simulink model "test_TM1654P"  (R2018b)
settings: Solver=FixedStepAuto  StartTime=0.0  StopTime=30  FixedStep=0.001  RelTol=1e-3
libraries: dspsrcs4 x1
settings Model: Creator=39926  LastModifiedBy=39926

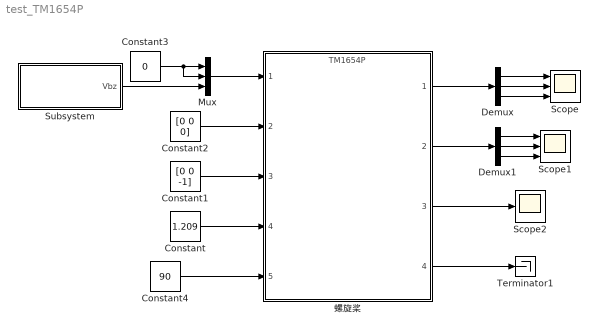
== system test_TM1654P ==
  Constant : Constant  Value=1.209  SampleTime=0
  Constant1 : Constant  Value=[0 0 -1]  SampleTime=0
  Constant2 : Constant  Value=[0 0 0]  SampleTime=0
  Constant3 : Constant  Value=0
  Constant4 : Constant  Value=90
  Demux : Demux  Outputs=3
  Demux1 : Demux  Outputs=3
  Mux : Mux  Inputs=3
  Scope : Scope  NumInputPorts=3
  Scope1 : Scope  NumInputPorts=3
  Scope2 : Scope
  Subsystem : Subsystem
  Terminator1 : Terminator
  螺旋桨 : ModelReference  ModelNameDialog=TM1654P  SimulationMode=Normal  ModelReferenceVersion=1.89
  wires:
  Mux/1 -> 螺旋桨/1
  Constant2/1 -> 螺旋桨/2
  Constant1/1 -> 螺旋桨/3
  Constant/1 -> 螺旋桨/4
  螺旋桨/1 -> Demux/1
  螺旋桨/2 -> Demux1/1
  Constant4/1 -> 螺旋桨/5
  螺旋桨/3 -> Scope2/1
  螺旋桨/4 -> Terminator1/1
  Demux/1 -> Scope/1
  Demux/2 -> Scope/2
  Demux/3 -> Scope/3
  Demux1/1 -> Scope1/1
  Demux1/2 -> Scope1/2
  Demux1/3 -> Scope1/3
  Subsystem/1("Vbz ") -> Mux/3
  Constant3/1 -> Mux/2, Mux/1

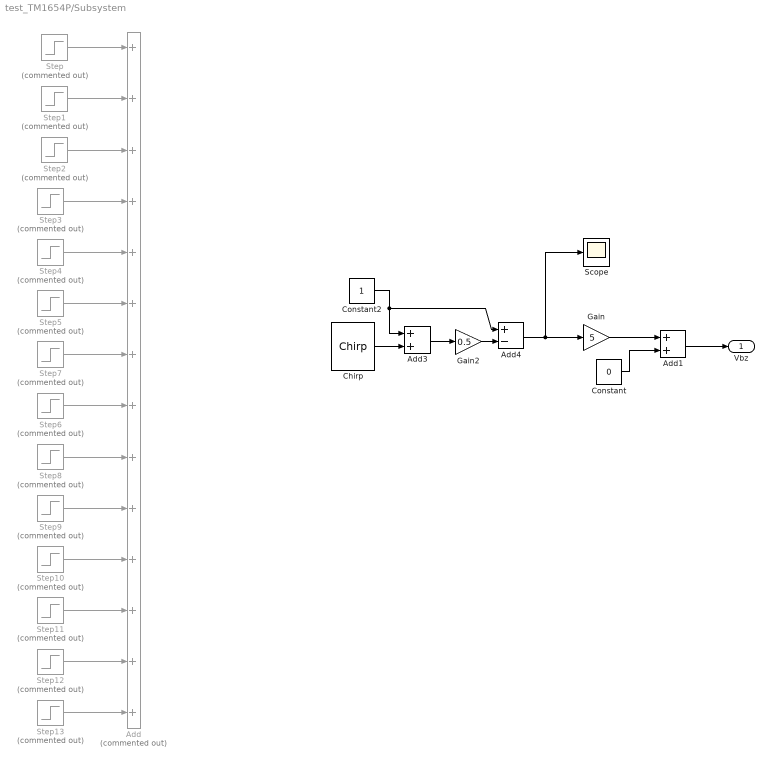
== system test_TM1654P/Subsystem ==
  Add : Sum  Commented=on  Inputs=++++++++++++++
  Add1 : Sum
  Add3 : Sum
  Add4 : Sum  Inputs=+-
  Chirp : dspsrcs4/Chirp  sweep=Linear  mode=Unidirectional  f0=0.1  f1=4  t1=30  Tsweep=30  phase=0  Ts=1/1000  spf=1  datatype=Double  OutputFrames=off
      settings: SourceProductName=DSP System Toolbox
  Constant : Constant  Value=0
  Constant2 : Constant
  Gain : Gain  Gain=5
  Gain2 : Gain  Gain=0.5
  Scope : Scope
  Step : Step  Commented=on  Time=2  After=1/14  SampleTime=0
  Step1 : Step  Commented=on  Time=4  After=1/14  SampleTime=0
  Step10 : Step  Commented=on  Time=22  After=1/14  SampleTime=0
  Step11 : Step  Commented=on  Time=24  After=1/14  SampleTime=0
  Step12 : Step  Commented=on  Time=26  After=1/14  SampleTime=0
  Step13 : Step  Commented=on  Time=28  After=1/14  SampleTime=0
  Step2 : Step  Commented=on  Time=6  After=1/14  SampleTime=0
  Step3 : Step  Commented=on  Time=8  After=1/14  SampleTime=0
  Step4 : Step  Commented=on  Time=10  After=1/14  SampleTime=0
  Step5 : Step  Commented=on  Time=12  After=1/14  SampleTime=0
  Step6 : Step  Commented=on  Time=16  After=1/14  SampleTime=0
  Step7 : Step  Commented=on  Time=14  After=1/14  SampleTime=0
  Step8 : Step  Commented=on  Time=18  After=1/14  SampleTime=0
  Step9 : Step  Commented=on  Time=20  After=1/14  SampleTime=0
  "Vbz " : Outport
  wires:
  Step/1 -> Add/1
  Step1/1 -> Add/2
  Step2/1 -> Add/3
  Step3/1 -> Add/4
  Step4/1 -> Add/5
  Step5/1 -> Add/6
  Step6/1 -> Add/8
  Gain/1 -> Add1/1
  Constant/1 -> Add1/2
  Add1/1 -> "Vbz "/1
  Step7/1 -> Add/7
  Step8/1 -> Add/9
  Step9/1 -> Add/10
  Step10/1 -> Add/11
  Step11/1 -> Add/12
  Step12/1 -> Add/13
  Step13/1 -> Add/14
  Chirp/1 -> Add3/2
  Constant2/1 -> Add4/1, Add3/1
  Add3/1 -> Gain2/1
  Gain2/1 -> Add4/2
  Add4/1 -> Scope/1, Gain/1
